simulink model "configurable_pwm"  (R2017a)
settings: Solver=VariableStepAuto  StartTime=0.0  StopTime=2000  RelTol=1e-3
libraries: hdlsllib x2
settings Model: Creator=wachala.j  LastModifiedBy=wachala.j

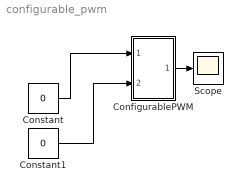
== system configurable_pwm ==
  ConfigurablePWM : Subsystem
  Constant : Constant  Value=0  OutDataTypeStr=boolean
  Constant1 : Constant  Value=0  OutDataTypeStr=boolean
  Scope : Scope
  wires:
  Constant/1 -> ConfigurablePWM/1(Enable)
  Constant1/1 -> ConfigurablePWM/2(Direction)
  ConfigurablePWM/1(PWM) -> Scope/1

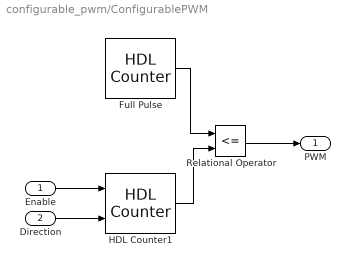
== system configurable_pwm/ConfigurablePWM ==
  Enable : Inport  OutDataTypeStr=boolean
  Direction : Inport  Port=2  OutDataTypeStr=boolean
  Full Pulse : hdlsllib/HDL Operations/HDL Counter  CountType=Count limited  CountInit=0  CountStep=1  CountMax=1000  CountFromType=Initial value  CountFrom=0  CountResetPort=off  CountLoadPort=off  CountEnbPort=off  CountDirPort=off  CountDataType=Unsigned  CountWordLen=32  CountFracLen=0  CountSampTime=1
      settings: SourceProductName=HDL Coder  SourceProductBaseCode=HD
  HDL Counter1 : hdlsllib/HDL Operations/HDL Counter  CountType=Count limited  CountInit=30  CountStep=6  CountMax=120  CountFromType=Initial value  CountFrom=30  CountResetPort=off  CountLoadPort=off  CountEnbPort=on  CountDirPort=on  CountDataType=Unsigned  CountWordLen=8  CountFracLen=0  CountSampTime=1
      settings: SourceProductName=HDL Coder  SourceProductBaseCode=HD
  Relational Operator : RelationalOperator  Operator=<=  OutDataTypeStr=boolean  RndMeth=Simplest
  PWM : Outport
  wires:
  Relational Operator/1 -> PWM/1
  HDL Counter1/1 -> Relational Operator/2
  Direction/1 -> HDL Counter1/2
  Full Pulse/1 -> Relational Operator/1
  Enable/1 -> HDL Counter1/1
